simulink model "satellite_sim"  (R2016b)
settings: Solver=ode45  StartTime=0.0  StopTime=200  RelTol=1e-3  EnableMultiTasking=on
InitFcn:
  | addpath ./..
  | satelliteParam
  | satelliteParamHW13
undefined symbols (not defined in the file or in its folder): P, satellite_animation, satellite_ctrl
settings Model: Creator=beard  LastModifiedBy=beard
settings DataIOCC: LimitDataPoints=on  SaveFormat=Array  SignalLoggingSaveFormat=ModelDataLogs
settings OptimizationCC: ExpressionDepthLimit=2147483647  InitFltsAndDblsToZero=on  LifeSpan=inf
settings DebuggingCC: UnderspecifiedInitializationDetection=Classic  MergeDetectMultiDrivingBlocksExec=none  SolverPrmCheckMsg=warning  FcnCallInpInsideContextMsg=warning  StateNameClashWarn=warning  SFUnexpectedBacktrackingDiag=warning  SFNoUnconditionalDefaultTransitionDiag=warning  SFExecutionAtInitializationDiag=none
settings HardwareCC: ProdBitPerPointer=32  ProdBitPerSizeT=32  ProdBitPerPtrDiffT=32  ProdLargestAtomicFloat=None  ProdIntDivRoundTo=Undefined  ProdEndianess=Unspecified  ProdWordSize=32  ProdHWDeviceType=32-bit Generic
settings ModelReferenceCC: PropagateSignalLabelsOutOfModel=off
settings GRTTargetCC: TargetLangStandard=C89/C90 (ANSI)  GeneratePreprocessorConditionals=Disable all  CombineOutputUpdateFcns=off  GRTInterface=on
settings ConfigComp: CovMetricSettings=dw  CovHtmlReporting=on  CovSaveCumulativeToWorkspaceVar=on  CovSaveSingleToWorkspaceVar=on  CovExternalEMLEnable=off

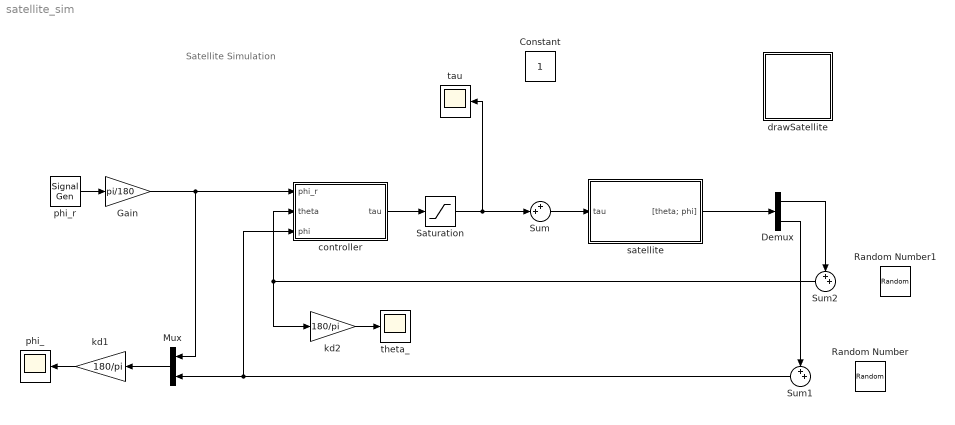
== system satellite_sim ==
  note: Satellite Simulation
  Constant : Constant
  Demux : Demux  Outputs=2
  Gain : Gain  Gain=pi/180
  Mux : Mux  Inputs=2
  Random Number : RandomNumber  Variance=.001^2  SampleTime=0.1
  Random Number1 : RandomNumber  Variance=.001^2  SampleTime=0.1
  Saturation : Saturate  UpperLimit=P.taumax  LowerLimit=-P.taumax
  Sum : Sum  Inputs=++|
  Sum1 : Sum  Inputs=++|
  Sum2 : Sum  Inputs=++|
  controller : Subsystem
  drawSatellite : Subsystem
      mask Display: image(imread('tv.jpg'))
  kd1 : Gain  Gain=180/pi
  kd2 : Gain  Gain=180/pi
  phi_ : Scope
  phi_r : SignalGenerator  WaveForm=square  Amplitude=15  Frequency=.02
  satellite : Subsystem
  tau : Scope
  theta_ : Scope
  wires:
  phi_r/1 -> Gain/1
  controller/1(tau) -> Saturation/1
  Gain/1 -> Mux/1, controller/1("phi_r  ")
  kd2/1 -> theta_/1
  Mux/1 -> kd1/1
  kd1/1 -> phi_/1
  Saturation/1 -> tau/1, Sum/2
  satellite/1("[theta; phi]") -> Demux/1
  Sum/1 -> satellite/1(tau)
  Demux/1 -> Sum2/1
  Demux/2 -> Sum1/1
  Sum1/1 -> controller/3(phi), Mux/2
  Sum2/1 -> kd2/1, controller/2(theta)

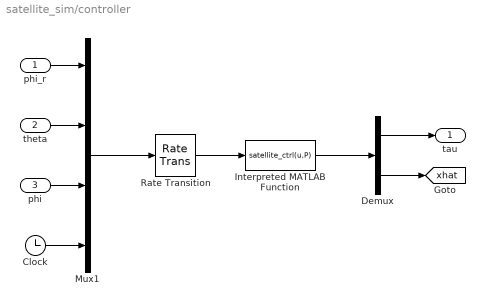
== system satellite_sim/controller ==
  "phi_r  " : Inport
  theta : Inport  Port=2
  phi : Inport  Port=3
  Clock : Clock
  Demux : Demux  Outputs=[1;4]
  Interpreted MATLAB Function : MATLABFcn  MATLABFcn=satellite_ctrl(u,P)  OutputDimensions=1+4
  Mux1 : Mux
  Rate Transition : RateTransition  OutPortSampleTime=P.Ts
  tau : Outport
  tag scope: xhat=global
  wires:
  Mux1/1 -> Rate Transition/1
  "phi_r  "/1 -> Mux1/1
  Clock/1 -> Mux1/4
  Rate Transition/1 -> Interpreted MATLAB Function/1
  phi/1 -> Mux1/3
  theta/1 -> Mux1/2
  Interpreted MATLAB Function/1 -> Demux/1
  Demux/1 -> tau/1
  Demux/2 -> [xhat]

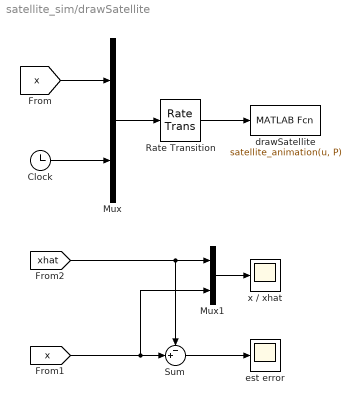
== system satellite_sim/drawSatellite ==
  Clock : Clock
  Mux : Mux  Inputs=2
  Mux1 : Mux  Inputs=2
  Rate Transition : RateTransition  OutPortSampleTime=P.t_plot
  Sum : Sum  Inputs=-+|
  drawSatellite : MATLABFcn  MATLABFcn=satellite_animation(u, P)  OutputDimensions=0
  est error : Scope
  x / xhat : Scope
  wires:
  [x] -> Sum/2, Mux1/2
  [xhat] -> Sum/1, Mux1/1
  Sum/1 -> est error/1
  Mux1/1 -> x / xhat/1
  Rate Transition/1 -> drawSatellite/1
  Clock/1 -> Mux/2
  [x] -> Mux/1
  Mux/1 -> Rate Transition/1

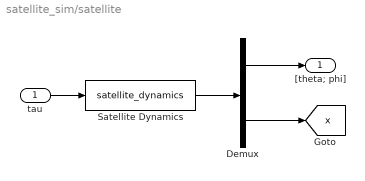
== system satellite_sim/satellite ==
  tau : Inport
  Demux : Demux  Outputs=[2;4]
  Satellite Dynamics : S-Function  FunctionName=satellite_dynamics  Parameters=P  SFunctionDeploymentMode=off  EnableBusSupport=off
  "[theta; phi]" : Outport
  tag scope: x=global
  wires:
  tau/1 -> Satellite Dynamics/1
  Satellite Dynamics/1 -> Demux/1
  Demux/1 -> "[theta; phi]"/1
  Demux/2 -> [x]
